simulink model "adaptive_thresholding_v2"  (R2024a)
settings: Solver=VariableStepAuto  StartTime=0.0  StopTime=10.0  RelTol=1e-3
undefined symbols (not defined in the file): xlfda_numerator
libraries: hdlBasic x12, hdlUtilities x1, commchan3 x1, dspsrcs4 x1, embmathops x1, dspmlti4 x1, vmcUtilities x1
settings Model: Creator=scorp  LastModifiedBy=saqib

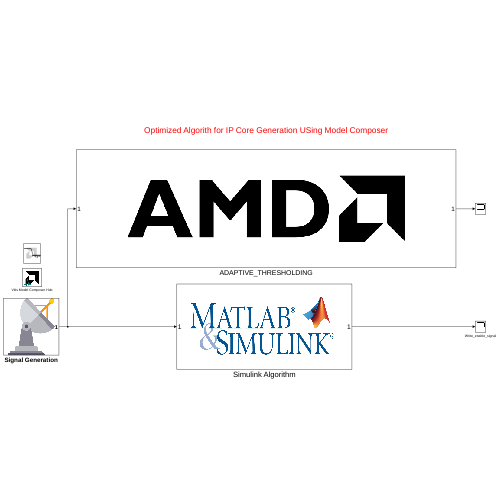
[thumbnail: Simulink's stored preview of the top-level diagram]
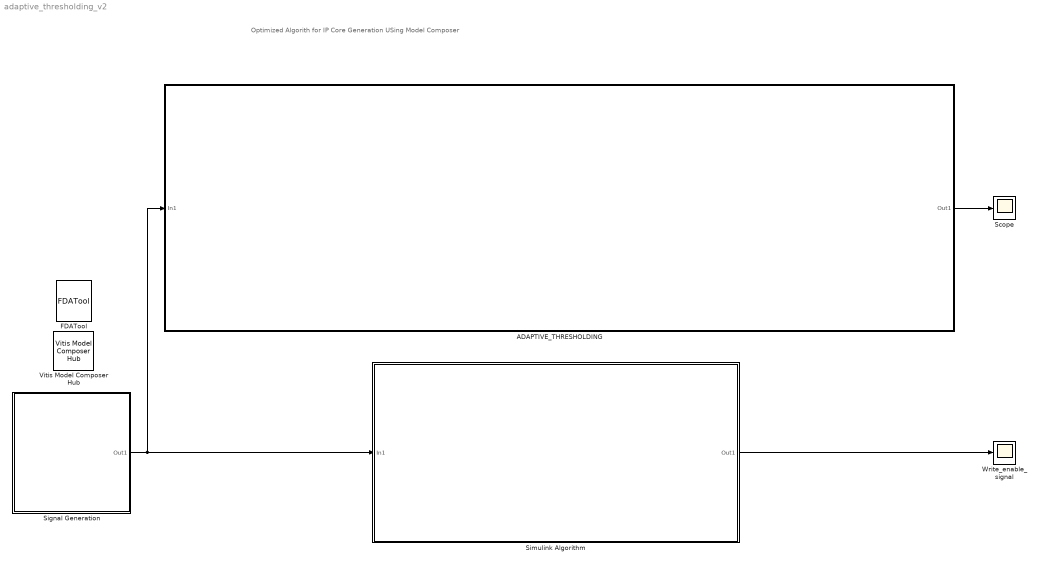
== system adaptive_thresholding_v2 ==
  note: Optimized Algorith for IP Core Generation USing Model Composer
  ADAPTIVE_THRESHOLDING : Subsystem
  FDATool : hdlUtilities/FDATool  block_type=fdatool
      settings: infoedit=FDATool
  Scope : Scope
  Signal Generation : Subsystem
      mask Display: image('124550.png');
  Simulink Algorithm : Subsystem
      mask Display: image('mlsl-12062018.jpg');
  Vitis Model Composer Hub : vmcUtilities/Vitis Model Composer Hub  Tag=genX  CodeGeneration=off  SubsystemName=ADAPTIVE_THRESHOLDING  CompilationType=HDLCompilation  SubsystemType=HDLNode  ExportTypeV2=IP Catalog  StartColumn=1  NumberOfColumns=1  TargetDirectory=/home/saqib/Desktop/resources/EW/Parameter_Estimation/MATLAB/DRIVE/Adpative_thresholding/HDL  exportDesign=on  analyzeDesign=off  validateDesignOnHw=off  ExportType=AI Engines  IpVendor=xilinx.com  IpLibrary=hls  IpVersion=1.0  IpHWLanguage=Verilog  AieCompilerOptions={}  AieSimulatorOptions={}  CreateTestbench=on  TestbenchStackSize=10  RunRtlSim=off  RunCSim=off  RunAieSim=off  AieSimTimeout=50000  RunAieSimProfiling=off  LaunchVitisAnalyzer=off  PlotOutput=off  RunX86Sim=off  X86SimTimeout=10  GenHwImage=off  GenLibadfXo=on  GenHwValidationCode=off  PlatformType=Not Specified  HwSystemType=Baremetal  HwValidationTarget=hw  ProjDevice=Zynq UltraScale+ ZCU102 Evaluation Board (xczu9eg-ffvb1156-2-e)  ProjDevicePart=xczu9eg-ffvb1156-2-e  AIEType=None  SamplePeriod=-1  ClockFrequency=200  DataPathParallelism=1  xilinxfamily=zynquplus  part=xczu9eg  speed=-2-e  package=ffvb1156  directory=<binary blob, 121 chars, not shown>  testbench=on  incr_netlist=off  synthesis_tool=Vivado  clock_wrapper=Clock Enables  dbl_ovrd=According to Block Masks  dcm_input_clock_period=10  sysclk_period=4  simulink_period=1/60e4  eval_field=0  IPInfoJsonString="{\"HDLSubsystem\":{\"SubsystemName\":\"ADAPTIVE_THRESHOLDING\",\"IPName\":\"IP\",\"IPLibrary\":\"VMC\",\"IPVendor\":\"User Company\",\"IPVersion\":\"1.0\",\"TargetDirectory\":\"/home/saqib/Desktop/resources/EW/Parameter_Estimation/MATLAB/DRIVE/Adpative_thresholding/HDL\",\"SubsystemDir\":\"/home/saqib/Desktop/resources/EW/Parameter_Estimation/MATLAB/DRIVE/Adpative_thresholding/HDL/ip/ADAPTIVE_THRESHOLDING\"}}"  LogFileName=/home/saqib/Desktop/resources/EW/Parameter_Estimation/MATLAB/DRIVE/Adpative_thresholding/HDL/model_composer.log  NThreads=4  IPConfigFile=/tmp/vmctmp-saqib/36106/ipconfig.json
  Write_enable_signal : Scope
  wires:
  Simulink Algorithm/1(Out1) -> Write_enable_signal/1
  ADAPTIVE_THRESHOLDING/1(Out1) -> Scope/1
  Signal Generation/1(Out1) -> Simulink Algorithm/1(In1), ADAPTIVE_THRESHOLDING/1(In1)

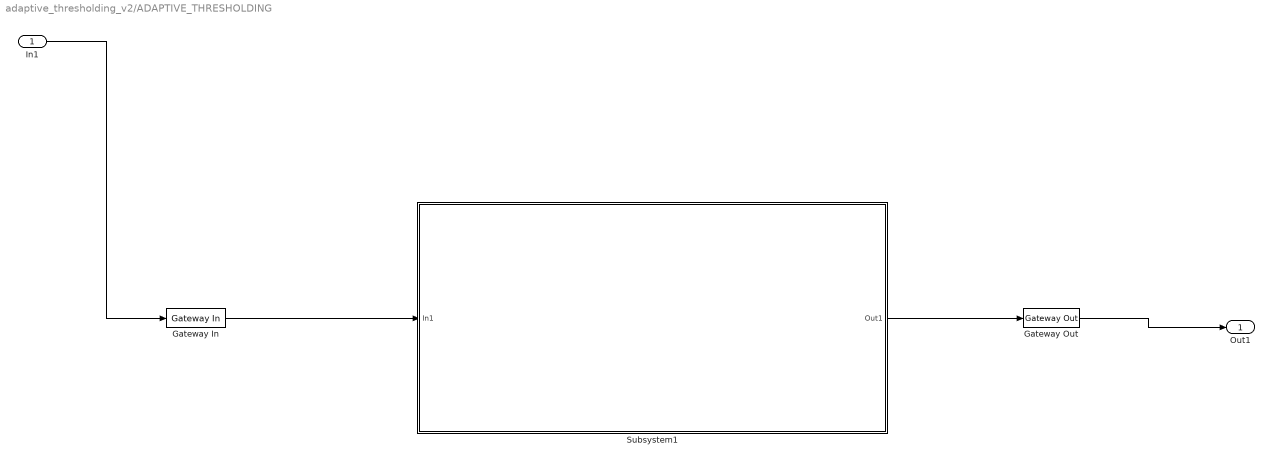
== system adaptive_thresholding_v2/ADAPTIVE_THRESHOLDING ==
  In1 : Inport
  Gateway In : hdlBasic/Gateway In  gui_display_data_type=Fixed-point  arith_type=Signed (2's comp)  n_bits=20  bin_pt=16  preci_type=Single  exp_width=8  frac_width=24  rows=1  columns=1  quantization="Round  (unbiased: +/- Inf)"  overflow=Saturate  period=1/60e4  UseAsADC=off  ADCChannel='1'  interface=None  automatic_assignment=on  address_offset=hex2dec('00')  intf_name=''  intf_description=''  default_value=0  timing_constraint=None  locs_specified=off  LOCs={}  io_standard={}  inherit_from_input=off  hdl_port=on  XmcBlockStatus=1  maskContainerNames=group4  block_type=gatewayin  block_config=sysgen:gateway_in_config  block_width_w=590  block_height_w=620  block_width=640  block_height=850
  Gateway Out : hdlBasic/Gateway Out  inherit_from_input=off  hdl_port=on  rows=1  columns=1  UseAsDAC=off  DACChannel='1'  interface=None  automatic_assignment=on  address_offset=hex2dec('00')  intf_name=''  intf_description=''  timing_constraint=None  locs_specified=off  LOCs={}  io_standard={}  XmcBlockStatus=1  maskContainerNames=group4  block_type=gatewayout  block_config=sysgen:gateway_out_config  block_width_w=590  block_height_w=620  block_width=620  block_height=750
  Subsystem1 : Subsystem
      mask Display: %%
  Out1 : Outport
  wires:
  Gateway In/1 -> Subsystem1/1(In1)
  Subsystem1/1(Out1) -> Gateway Out/1
  Gateway Out/1 -> Out1/1
  In1/1 -> Gateway In/1

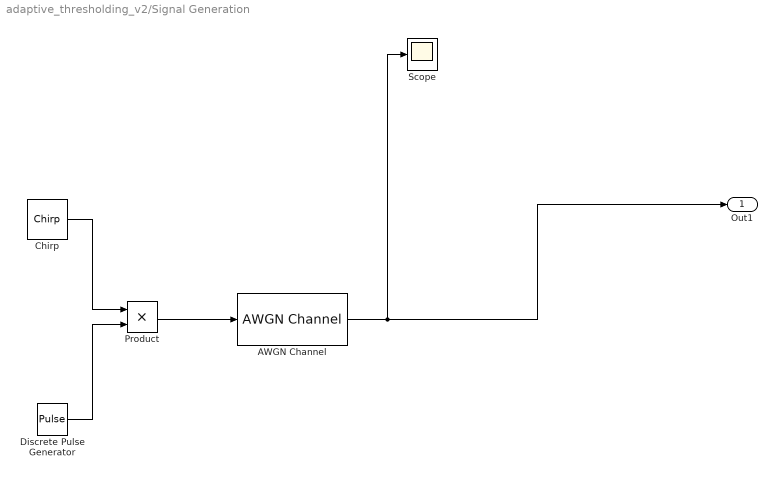
== system adaptive_thresholding_v2/Signal Generation ==
  AWGN Channel : commchan3/AWGN Channel  LegacyMode=off  NoiseMethod="Signal to noise ratio  (SNR)"  noiseMode="Signal to noise ratio  (SNR)"  EbNo=10  EsNo=10  SNR=7  BitsPerSymbol=1  SignalPower=1  SamplesPerSymbol=1  SymbolPeriod=1  VarianceSource=Parameter  Variance=1  RandomStream=Global stream  Seed=67  SimulateUsing=Code generation
  Chirp : dspsrcs4/Chirp  sweep=Linear  mode=Unidirectional  f0=30e3  f1=60e3  t1=10e-3  Tsweep=10e-3  phase=0  Ts=1/60e4  spf=1  datatype=double  OutputFrames=off
  Discrete Pulse Generator : DiscretePulseGenerator  Period=1*(60e4)  PulseWidth=100e-3*(60e4)  PhaseDelay=1*(60e4)  SampleTime=1/60e4
  Product : Product
  Scope : Scope
  Out1 : Outport
  wires:
  Chirp/1 -> Product/1
  Product/1 -> AWGN Channel/1
  Discrete Pulse Generator/1 -> Product/2
  AWGN Channel/1 -> Scope/1, Out1/1

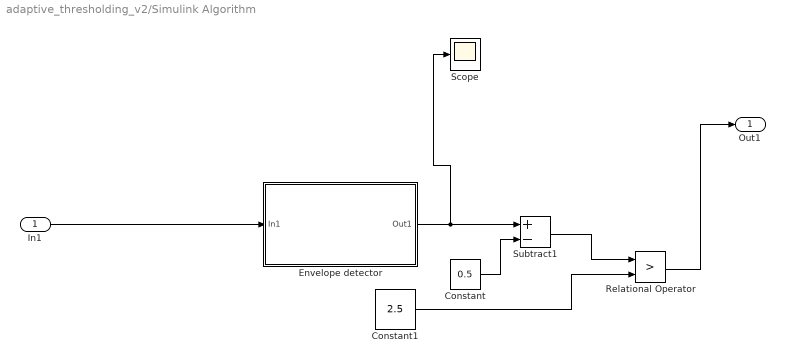
== system adaptive_thresholding_v2/Simulink Algorithm ==
  In1 : Inport
  Constant : Constant  Value=0.5
  Constant1 : Constant  Value=2.5  VectorParams1D=off  SampleTime=-1
  Envelope detector : Subsystem
  Relational Operator : RelationalOperator  Operator=>  OutDataTypeStr=boolean  RndMeth=Zero  InputSameDT=off
  Scope : Scope
  Subtract1 : Sum  Inputs=+-
  Out1 : Outport
  wires:
  In1/1 -> Envelope detector/1(In1)
  Constant/1 -> Subtract1/2
  Constant1/1 -> Relational Operator/2
  Subtract1/1 -> Relational Operator/1
  Envelope detector/1(Out1) -> Scope/1, Subtract1/1
  Relational Operator/1 -> Out1/1

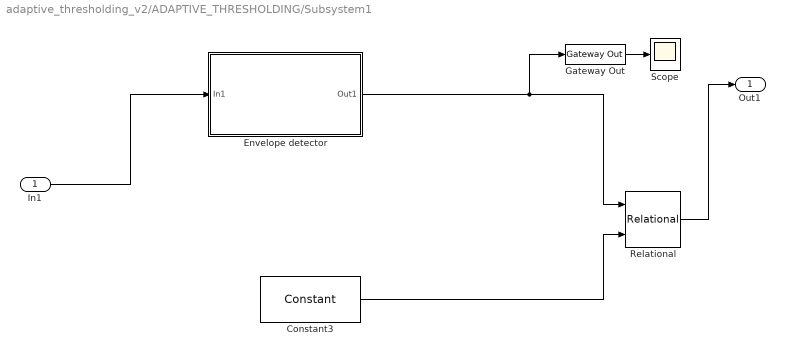
== system adaptive_thresholding_v2/ADAPTIVE_THRESHOLDING/Subsystem1 ==
  In1 : Inport
  Constant3 : hdlBasic/Constant  const=2.5  gui_display_data_type=Fixed-point  arith_type=Signed (2's comp)  n_bits=20  bin_pt=14  preci_type=Single  exp_width=8  frac_width=24  explicit_period=off  period=1  XmcBlockStatus=1  maskContainerNames=tabcontainer1  block_type=constant  block_config=sysgen:Constant_config
  Envelope detector : Subsystem
  Gateway Out : hdlBasic/Gateway Out  inherit_from_input=off  hdl_port=off  rows=1  columns=1  UseAsDAC=off  DACChannel='1'  interface=None  automatic_assignment=on  address_offset=hex2dec('00')  intf_name=''  intf_description=''  timing_constraint=None  locs_specified=off  LOCs={}  io_standard={}  XmcBlockStatus=1  maskContainerNames=group4  block_type=gatewayout  block_config=sysgen:gateway_out_config  block_width_w=590  block_height_w=620  block_width=620  block_height=750
  Relational : hdlBasic/Relational  mode=a>b  op_type=Bool  en=off  latency=1  XmcBlockStatus=1  maskContainerNames=tabcontainer1  block_type=relational  block_config=sysgen:Relational_config
  Scope : Scope
  Out1 : Outport
  wires:
  Relational/1 -> Out1/1
  Constant3/1 -> Relational/2
  In1/1 -> Envelope detector/1(In1)
  Envelope detector/1(Out1) -> Gateway Out/1, Relational/1
  Gateway Out/1 -> Scope/1

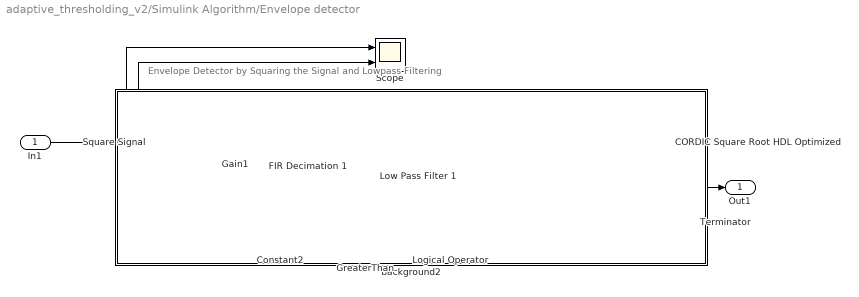
== system adaptive_thresholding_v2/Simulink Algorithm/Envelope detector ==
  note: Envelope Detector by Squaring the Signal and Lowpass Filtering
  In1 : Inport
  CORDIC Square Root HDL Optimized : embmathops/CORDIC Square Root HDL Optimized  autoMaximumShiftVal=on  maximumShiftValue=10  nIterPerReg=1
      settings: LibrarySourceBlock=embeddedMatrixLib/Math Operations/CORDIC Square Root HDL Optimized
  Constant2 : Constant
  FIR Decimation 1 : dspmlti4/FIR Decimation  FilterSource=Dialog parameters  h=[1 1 1 1 1]  D=10  filtStruct=Direct form  FilterObject=Hm_firdecim  InputProcessing=Columns as channels (frame based)  framing=Allow multirate processing  AllowArbitraryInputLength=off  inputOffset=0  outputBufInitCond=0  roundingMode=Floor  overflowMode=off  firstCoeffDataTypeStr=Inherit: Same word length as input  firstCoeffMin=[]  firstCoeffMax=[]  firstCoeffLastDataTypeStr=Inherit: Same word length as input  outputMin=[]  outputMax=[]
  Gain1 : Gain  Gain=4
  GreaterThan : RelationalOperator  Operator===  OutDataTypeStr=boolean  RndMeth=Simplest  InputSameDT=off
  Logical Operator : Logic  Operator=NOT  AllPortsSameDT=off  OutDataTypeStr=boolean
  Low Pass Filter 1 : DiscreteFir  Coefficients=firpm(20, [0 0.03 0.1 1], [1 1 0 0])  InputProcessing=Columns as channels (frame based)  AccumDataTypeStr=Inherit: Same as product output
  Scope : Scope  NumInputPorts=2
  Square Signal : Math  Operator=square  SignedPower=on
  Terminator : Terminator
  background2 : Subsystem
      mask Display: disp('')
  Out1 : Outport
  wires:
  Square Signal/1 -> Gain1/1
  Gain1/1 -> Scope/2, FIR Decimation 1/1
  In1/1 -> Square Signal/1
  FIR Decimation 1/1 -> Scope/1, Low Pass Filter 1/1
  Low Pass Filter 1/1 -> CORDIC Square Root HDL Optimized/1
  CORDIC Square Root HDL Optimized/1 -> Out1/1
  GreaterThan/1 -> CORDIC Square Root HDL Optimized/2, Logical Operator/1
  Constant2/1 -> GreaterThan/2, GreaterThan/1
  Logical Operator/1 -> CORDIC Square Root HDL Optimized/3
  CORDIC Square Root HDL Optimized/2 -> Terminator/1

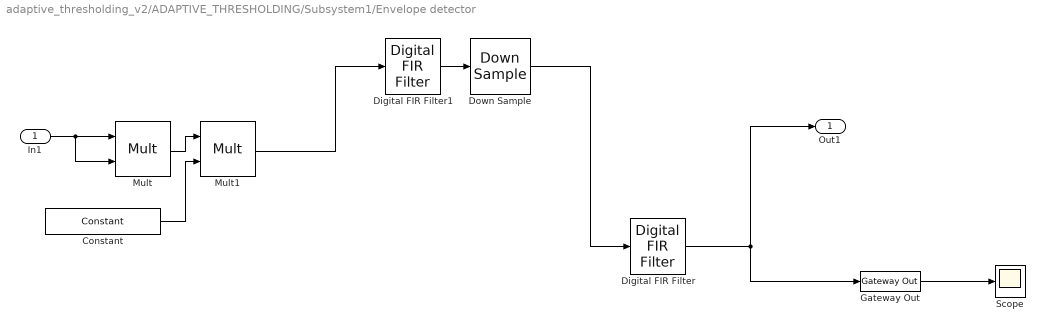
== system adaptive_thresholding_v2/ADAPTIVE_THRESHOLDING/Subsystem1/Envelope detector ==
  In1 : Inport
  Constant : hdlBasic/Constant  const=4  gui_display_data_type=Fixed-point  arith_type=Unsigned  n_bits=20  bin_pt=14  preci_type=Single  exp_width=8  frac_width=24  explicit_period=off  period=1  XmcBlockStatus=1  maskContainerNames=tabcontainer1  block_type=constant  block_config=sysgen:Constant_config
  Digital FIR Filter : hdlBasic/Digital FIR Filter  coeff_source=off  coefficientvector=firpm(20, [0 0.03 0.1 1], [1 1 0 0])  coeff_calulate=off  coefficient_width=30  coefficient_fractional_bits=20  interpolation_filter_rate=1  decimation_filter_rate=1  fda_coefficientvector=[-0.0024 -0.0042 0.0095 0.0200 -0.0380 -0.0696 0.1374 0.4472 0.4472 0.1374 -0.0696 -0.0380 0.0200 0.0095 -0.0042 -0.0024]  simulation_type=fast_sim  simulation_model=sysgen:fir_macro  XmcBlockStatus=1  maskContainerNames=group1  block_type=fir_macro  block_config=sysgen:fir_macro_config
  Digital FIR Filter1 : hdlBasic/Digital FIR Filter  coeff_source=off  coefficientvector=xlfda_numerator( [bdroot, '/FDATool'])  coeff_calulate=on  coefficient_width=2  coefficient_fractional_bits=2  interpolation_filter_rate=1  decimation_filter_rate=1  fda_coefficientvector=[0.232365178390872 0.352783272606701 0.352783272606701 0.232365178390872]  simulation_type=fast_sim  simulation_model=sysgen:fir_macro  XmcBlockStatus=1  maskContainerNames=group1  block_type=fir_macro  block_config=sysgen:fir_macro_config
  Down Sample : hdlBasic/Down Sample  sample_ratio=10  sample_phase="Last Value of Frame  (most efficient)"  en=off  rst=off  latency=1  XmcBlockStatus=1  maskContainerNames=group1  block_type=dsamp  block_config=sysgen:Downsample_config
  Gateway Out : hdlBasic/Gateway Out  inherit_from_input=off  hdl_port=off  rows=1  columns=1  UseAsDAC=off  DACChannel='1'  interface=None  automatic_assignment=on  address_offset=hex2dec('00')  intf_name=''  intf_description=''  timing_constraint=None  locs_specified=off  LOCs={}  io_standard={}  XmcBlockStatus=1  maskContainerNames=group4  block_type=gatewayout  block_config=sysgen:gateway_out_config  block_width_w=590  block_height_w=620  block_width=620  block_height=750
  Mult : hdlBasic/Mult  precision=User Defined  arith_type=Unsigned  n_bits=30  bin_pt=20  quantization=Truncate  overflow=Wrap  en=off  latency=3  opt_float=off  fp_mult_usage=No Usage  use_behavioral_HDL=off  opt=Speed  use_embedded=on  optimum_pipeline=off  pipeline=on  use_rpm=on  placement_style=Triangular  XmcBlockStatus=1  maskContainerNames=group1  block_type=mult  block_config=sysgen:Mult_config  block_width=598  block_height=876
  Mult1 : hdlBasic/Mult  precision=User Defined  arith_type=Unsigned  n_bits=30  bin_pt=20  quantization=Truncate  overflow=Wrap  en=off  latency=3  opt_float=off  fp_mult_usage=No Usage  use_behavioral_HDL=off  opt=Speed  use_embedded=on  optimum_pipeline=off  pipeline=on  use_rpm=on  placement_style=Triangular  XmcBlockStatus=1  maskContainerNames=group1  block_type=mult  block_config=sysgen:Mult_config  block_width=598  block_height=876
  Scope : Scope
  Out1 : Outport
  wires:
  Mult1/1 -> Digital FIR Filter1/1
  In1/1 -> Mult/2, Mult/1
  Mult/1 -> Mult1/1
  Constant/1 -> Mult1/2
  Down Sample/1 -> Digital FIR Filter/1
  Digital FIR Filter1/1 -> Down Sample/1
  Digital FIR Filter/1 -> Out1/1, Gateway Out/1
  Gateway Out/1 -> Scope/1

== system adaptive_thresholding_v2/Simulink Algorithm/Envelope detector/background2 ==
